simulink model "Mo_phong_3"  (R2019a)
settings: Solver=FixedStepAuto  StartTime=0.0  StopTime=55  FixedStep=0.01  RelTol=1e-3
undefined symbols (not defined in the file): magnitude
libraries: mobileRoboticsLib x13, simulink x6
settings Model: Creator=chemi  LastModifiedBy=chemi

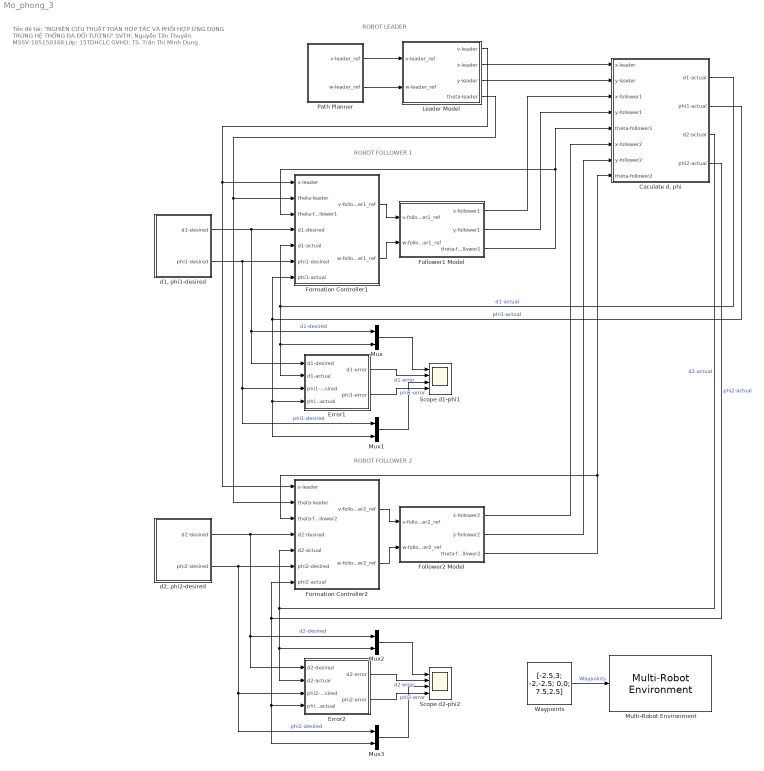
== system Mo_phong_3 ==
  note: ROBOT FOLLOWER 1
  note: ROBOT LEADER
  note: ROBOT FOLLOWER 2
  note: Tên đề tài: "NGHIÊN CỨU THUẬT TOÁN HỢP TÁC
      | VÀ PHỐI HỢP ỨNG DỤNG TRONG HỆ THỐNG
      | ĐA ĐỐI TƯỢNG"
      |
      | SVTH: Nguyễn Tấn Thuyền MSSV:105150348
      | Lớp: 15TDHCLC
      | GVHD: TS. Trần Thị Minh Dung
  "Caculate d, phi" : Subsystem
  Error1 : Subsystem
  Error2 : Subsystem
  Follower1 Model : Subsystem
  Follower2 Model : Subsystem
  Formation Controller1 : Subsystem
  Formation Controller2 : Subsystem
  Leader Model : Subsystem
  Multi-Robot Environment : mobileRoboticsLib/Environments/Multi-Robot Environment  numRobots=3  showWaypoints=on  showObjects=off  objectColors=[1 0 0;0 1 0;0 0 1]  objectMarkers='s'  showRobotIds=on  plotSensorLines=off
      settings: SourceProductName=Mobile Robotics Simulation Toolbox
  Mux{,1..3} (4 alike) : Mux  Inputs=2
  Path Planner : Subsystem
  Scope d1-phi1 : Scope  NumInputPorts=4
  Scope d2-phi2 : Scope  NumInputPorts=4
  Waypoints : Constant  Value=[-2.5,3; -2,-2.5; 0,0; 7.5,2.5]
  "d1, phi1-desired" : Subsystem
  "d2, phi2-desired" : Subsystem
  wires:
  Path Planner/1(v-leader_ref) -> Leader Model/1(v-leader_ref)
  Leader Model/2(x-leader) -> "Caculate d, phi"/1(x-leader)
  Follower1 Model/2(y-follower1) -> "Caculate d, phi"/4(y-follower1)
  Leader Model/3(y-leader) -> "Caculate d, phi"/2(y-leader)
  Follower1 Model/1(x-follower1) -> "Caculate d, phi"/3(x-follower1)
  Follower1 Model/3(theta-follower1) -> "Caculate d, phi"/5(theta-follower1), Formation Controller1/3(theta-follower1)
  "Caculate d, phi"/2(phi1-actual) -> Formation Controller1/7(phi1-actual), Mux1/2, Error1/4(phi1-actual)  "phi1-actual"
  "Caculate d, phi"/1(d1-actual) -> Formation Controller1/5(d1-actual), Mux/2, Error1/2(d1-actual)  "d1-actual"
  Leader Model/1(v-leader) -> Formation Controller1/1(v-leader), Formation Controller2/1(v-leader)
  Leader Model/4(theta-leader) -> Formation Controller1/2(theta-leader), Formation Controller2/2(theta-leader)
  "d1, phi1-desired"/2(phi1-desired) -> Mux1/1, Error1/3(phi1-desired), Formation Controller1/6(phi1-desired)  "phi1-desired"
  "d1, phi1-desired"/1(d1-desired) -> Mux/1, Error1/1(d1-desired), Formation Controller1/4(d1-desired)  "d1-desired"
  Formation Controller2/2(w-follower2_ref) -> Follower2 Model/2(w-follower2_ref)
  Follower2 Model/1(x-follower2) -> "Caculate d, phi"/6(x-follower2)
  Follower2 Model/2(y-follower2) -> "Caculate d, phi"/7(y-follower2)
  Follower2 Model/3(theta-follower2) -> "Caculate d, phi"/8(theta-follower2), Formation Controller2/3(theta-follower2)
  "Caculate d, phi"/3(d2-actual) -> Mux2/2, Error2/2(d2-actual), Formation Controller2/5(d2-actual)  "d2-actual"
  "Caculate d, phi"/4(phi2-actual) -> Formation Controller2/7(phi2-actual), Mux3/2, Error2/4(phi2-actual)  "phi2-actual"
  "d2, phi2-desired"/1(d2-desired) -> Mux2/1, Error2/1(d2-desired), Formation Controller2/4(d2-desired)  "d2-desired"
  "d2, phi2-desired"/2(phi2-desired) -> Mux3/1, Error2/3(phi2-desired), Formation Controller2/6(phi2-desired)  "phi2-desired"
  Waypoints/1 -> Multi-Robot Environment/1  "Waypoints"
  Path Planner/2(w-leader_ref) -> Leader Model/2(w-leader_ref)
  Formation Controller1/1(v-follower1_ref) -> Follower1 Model/1(v-follower1_ref)
  Formation Controller1/2(w-follower1_ref) -> Follower1 Model/2(w-follower1_ref)
  Formation Controller2/1(v-follower2_ref) -> Follower2 Model/1(v-follower2_ref)
  Mux/1 -> Scope d1-phi1/1
  Error1/1(d1-error) -> Scope d1-phi1/2  "d1-error"
  Mux1/1 -> Scope d1-phi1/3
  Error1/2(phi1-error) -> Scope d1-phi1/4  "phi1-error"
  Mux2/1 -> Scope d2-phi2/1
  Error2/1(d2-error) -> Scope d2-phi2/2  "d2-error"
  Mux3/1 -> Scope d2-phi2/3
  Error2/2(phi2-error) -> Scope d2-phi2/4  "phi2-error"

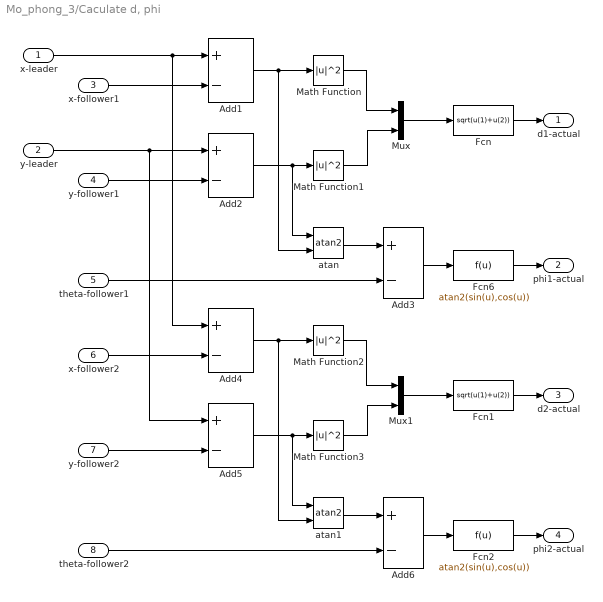
== system Mo_phong_3/Caculate d, phi ==
  x-leader : Inport
  y-leader : Inport  Port=2
  x-follower1 : Inport  Port=3
  y-follower1 : Inport  Port=4
  theta-follower1 : Inport  Port=5
  x-follower2 : Inport  Port=6
  y-follower2 : Inport  Port=7
  theta-follower2 : Inport  Port=8
  Add{1..6} (6 alike) : Sum  Inputs=+-
  Fcn : Fcn  Expr=sqrt(u(1)+u(2))
  Fcn1 : Fcn  Expr=sqrt(u(1)+u(2))
  Fcn2 : Fcn  Expr=atan2(sin(u),cos(u))
  Fcn6 : Fcn  Expr=atan2(sin(u),cos(u))
  Math Function{,1..3} (4 alike) : Math  Operator=magnitude^2  SaturateOnIntegerOverflow=on
  Mux : Mux  Inputs=2
  Mux1 : Mux  Inputs=2
  atan : Trigonometry  Operator=atan2
  atan1 : Trigonometry  Operator=atan2
  d1-actual : Outport
  phi1-actual : Outport  Port=2
  d2-actual : Outport  Port=3
  phi2-actual : Outport  Port=4
  wires:
  Math Function1/1 -> Mux/2
  Math Function/1 -> Mux/1
  Mux/1 -> Fcn/1
  Fcn/1 -> d1-actual/1
  Add2/1 -> atan/1, Math Function1/1
  Add1/1 -> atan/2, Math Function/1
  x-follower1/1 -> Add1/2
  y-follower1/1 -> Add2/2
  atan/1 -> Add3/1
  theta-follower1/1 -> Add3/2
  y-follower2/1 -> Add5/2
  y-leader/1 -> Add5/1, Add2/1
  x-follower2/1 -> Add4/2
  x-leader/1 -> Add4/1, Add1/1
  Add4/1 -> atan1/2, Math Function2/1
  Add5/1 -> atan1/1, Math Function3/1
  Fcn1/1 -> d2-actual/1
  Mux1/1 -> Fcn1/1
  Math Function2/1 -> Mux1/1
  Math Function3/1 -> Mux1/2
  atan1/1 -> Add6/1
  theta-follower2/1 -> Add6/2
  Add3/1 -> Fcn6/1
  Add6/1 -> Fcn2/1
  Fcn6/1 -> phi1-actual/1
  Fcn2/1 -> phi2-actual/1

== system Mo_phong_3/Error1 ==
  d1-desired : Inport
  d1-actual : Inport  Port=2
  phi1-desired : Inport  Port=3
  phi1-actual : Inport  Port=4
  Add2 : Sum  Inputs=+-
  Add3 : Sum  Inputs=+-
  d1-error : Outport
  phi1-error : Outport  Port=2
  wires:
  phi1-actual/1 -> Add3/2
  d1-actual/1 -> Add2/2
  phi1-desired/1 -> Add3/1
  d1-desired/1 -> Add2/1
  Add2/1 -> d1-error/1
  Add3/1 -> phi1-error/1

== system Mo_phong_3/Error2 ==
  d2-desired : Inport
  d2-actual : Inport  Port=2
  phi2-desired : Inport  Port=3
  phi2-actual : Inport  Port=4
  Add2 : Sum  Inputs=+-
  Add3 : Sum  Inputs=+-
  d2-error : Outport
  phi2-error : Outport  Port=2
  wires:
  phi2-actual/1 -> Add3/2
  d2-actual/1 -> Add2/2
  phi2-desired/1 -> Add3/1
  d2-desired/1 -> Add2/1
  Add2/1 -> d2-error/1
  Add3/1 -> phi2-error/1

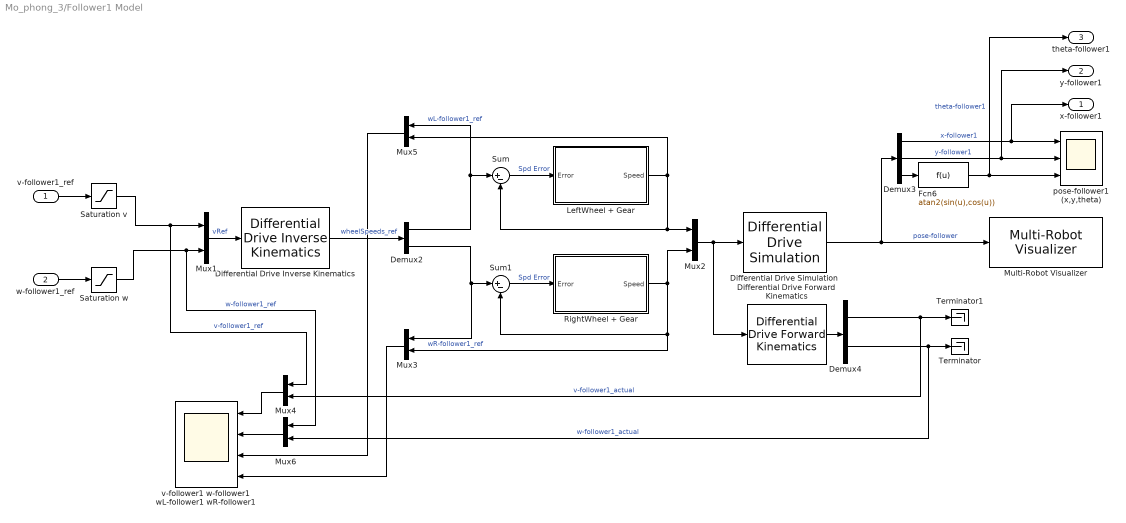
== system Mo_phong_3/Follower1 Model ==
  v-follower1_ref : Inport
  w-follower1_ref : Inport  Port=2
  Demux2 : Demux  Outputs=2
  Demux3 : Demux  Outputs=3
  Demux4 : Demux  Outputs=2
  Differential Drive Forward Kinematics : mobileRoboticsLib/Kinematic Models/Differential Drive/Differential Drive Forward Kinematics  wheelRadius=0.0425  wheelBase=0.25
      settings: SourceProductName=Mobile Robotics Simulation Toolbox
  Differential Drive Inverse Kinematics : mobileRoboticsLib/Kinematic Models/Differential Drive/Differential Drive Inverse Kinematics  wheelRadius=0.0425  wheelBase=0.25
      settings: SourceProductName=Mobile Robotics Simulation Library
  Differential Drive Simulation : mobileRoboticsLib/Kinematic Models/Differential Drive/Differential Drive Simulation  wheelRadius=0.0425  wheelBase=0.25  initX=-2.5  initY=3  initAngle=0  Ts=0.01
      settings: SourceProductName=Mobile Robotics Simulation Library
  Fcn6 : Fcn  Expr=atan2(sin(u),cos(u))
  LeftWheel + Gear : Subsystem
  Multi-Robot Visualizer : mobileRoboticsLib/Environments/Multi-Robot Visualizer  idx=2  radius=0.15  robotColor=[0.39 0.83 0.07]  showTraj=on  hasLidar=off  sensorOffset=[0,0]  scanAngles=[-pi/4, 0, pi/4]  hasObjDetector=off  objDetectorOffset=[0,0]  objDetectorAngle=0  objDetectorFOV=pi/3  objDetectorMaxRange=5
      settings: SourceProductName=Mobile Robotics Simulation Toolbox
  Mux{1..6} (6 alike) : Mux  Inputs=2
  RightWheel + Gear : Subsystem
  Saturation v : Saturate  UpperLimit=1  LowerLimit=0
  Saturation w : Saturate  UpperLimit=0.8  LowerLimit=-0.8
  Sum : Sum  Inputs=|+-
  Sum1 : Sum  Inputs=|+-
  Terminator : Terminator
  Terminator1 : Terminator
  pose-follower1 (x,y,theta) : Scope  NumInputPorts=3
  v-follower1 w-follower1 wL-follower1 wR-follower1 : Scope  NumInputPorts=4
  x-follower1 : Outport
  y-follower1 : Outport  Port=2
  theta-follower1 : Outport  Port=3
  wires:
  Demux3/2 -> pose-follower1 (x,y,theta)/2, y-follower1/1  "y-follower1"
  Differential Drive Simulation/1 -> Multi-Robot Visualizer/1, Demux3/1  "pose-follower"
  Demux3/3 -> Fcn6/1
  Differential Drive Inverse Kinematics/1 -> Demux2/1  "wheelSpeeds_ref"
  v-follower1_ref/1 -> Saturation v/1
  Demux3/1 -> pose-follower1 (x,y,theta)/1, x-follower1/1  "x-follower1"
  w-follower1_ref/1 -> Saturation w/1
  Mux1/1 -> Differential Drive Inverse Kinematics/1  "vRef"
  Demux2/2 -> Mux3/1, Sum1/1  "wR-follower1_ref"
  Demux2/1 -> Mux5/1, Sum/1  "wL-follower1_ref"
  Sum/1 -> LeftWheel + Gear/1(Error)  "Spd Error"
  LeftWheel + Gear/1(Speed) -> Mux2/1, Sum/2, Mux5/2
  Sum1/1 -> RightWheel + Gear/1(Error)  "Spd Error"
  RightWheel + Gear/1(Speed) -> Mux3/2, Sum1/2, Mux2/2
  Mux2/1 -> Differential Drive Simulation/1, Differential Drive Forward Kinematics/1
  Demux4/2 -> Mux6/2, Terminator/1  "w-follower1_actual"
  Differential Drive Forward Kinematics/1 -> Demux4/1
  Demux4/1 -> Terminator1/1, Mux4/2  "v-follower1_actual"
  Saturation v/1 -> Mux1/1, Mux4/1  "v-follower1_ref"
  Saturation w/1 -> Mux6/1, Mux1/2  "w-follower1_ref"
  Fcn6/1 -> pose-follower1 (x,y,theta)/3, theta-follower1/1  "theta-follower1"
  Mux4/1 -> v-follower1 w-follower1 wL-follower1 wR-follower1/1
  Mux6/1 -> v-follower1 w-follower1 wL-follower1 wR-follower1/2
  Mux5/1 -> v-follower1 w-follower1 wL-follower1 wR-follower1/3
  Mux3/1 -> v-follower1 w-follower1 wL-follower1 wR-follower1/4

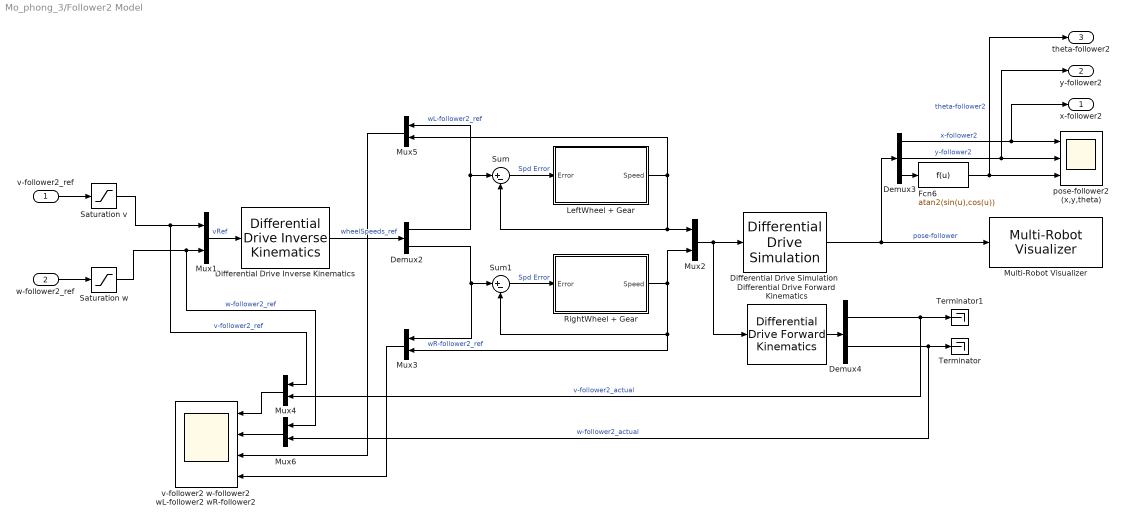
== system Mo_phong_3/Follower2 Model ==
  v-follower2_ref : Inport
  w-follower2_ref : Inport  Port=2
  Demux2 : Demux  Outputs=2
  Demux3 : Demux  Outputs=3
  Demux4 : Demux  Outputs=2
  Differential Drive Forward Kinematics : mobileRoboticsLib/Kinematic Models/Differential Drive/Differential Drive Forward Kinematics  wheelRadius=0.0425  wheelBase=0.25
      settings: SourceProductName=Mobile Robotics Simulation Toolbox
  Differential Drive Inverse Kinematics : mobileRoboticsLib/Kinematic Models/Differential Drive/Differential Drive Inverse Kinematics  wheelRadius=0.0425  wheelBase=0.25
      settings: SourceProductName=Mobile Robotics Simulation Library
  Differential Drive Simulation : mobileRoboticsLib/Kinematic Models/Differential Drive/Differential Drive Simulation  wheelRadius=0.0425  wheelBase=0.25  initX=-2  initY=-2.5  initAngle=0  Ts=0.01
      settings: SourceProductName=Mobile Robotics Simulation Library
  Fcn6 : Fcn  Expr=atan2(sin(u),cos(u))
  LeftWheel + Gear : Subsystem
  Multi-Robot Visualizer : mobileRoboticsLib/Environments/Multi-Robot Visualizer  idx=3  radius=0.15  robotColor=[0.00 0.45 0.74]  showTraj=on  hasLidar=off  sensorOffset=[0,0]  scanAngles=[-pi/4, 0, pi/4]  hasObjDetector=off  objDetectorOffset=[0,0]  objDetectorAngle=0  objDetectorFOV=pi/3  objDetectorMaxRange=5
      settings: SourceProductName=Mobile Robotics Simulation Toolbox
  Mux{1..6} (6 alike) : Mux  Inputs=2
  RightWheel + Gear : Subsystem
  Saturation v : Saturate  UpperLimit=1  LowerLimit=0
  Saturation w : Saturate  UpperLimit=0.8  LowerLimit=-0.8
  Sum : Sum  Inputs=|+-
  Sum1 : Sum  Inputs=|+-
  Terminator : Terminator
  Terminator1 : Terminator
  pose-follower2 (x,y,theta) : Scope  NumInputPorts=3
  v-follower2 w-follower2 wL-follower2 wR-follower2 : Scope  NumInputPorts=4
  x-follower2 : Outport
  y-follower2 : Outport  Port=2
  theta-follower2 : Outport  Port=3
  wires:
  Demux3/2 -> pose-follower2 (x,y,theta)/2, y-follower2/1  "y-follower2"
  Differential Drive Simulation/1 -> Multi-Robot Visualizer/1, Demux3/1  "pose-follower"
  Demux3/3 -> Fcn6/1
  Differential Drive Inverse Kinematics/1 -> Demux2/1  "wheelSpeeds_ref"
  v-follower2_ref/1 -> Saturation v/1
  Demux3/1 -> pose-follower2 (x,y,theta)/1, x-follower2/1  "x-follower2"
  w-follower2_ref/1 -> Saturation w/1
  Mux1/1 -> Differential Drive Inverse Kinematics/1  "vRef"
  Demux2/2 -> Mux3/1, Sum1/1  "wR-follower2_ref"
  Demux2/1 -> Mux5/1, Sum/1  "wL-follower2_ref"
  Sum/1 -> LeftWheel + Gear/1(Error)  "Spd Error"
  LeftWheel + Gear/1(Speed) -> Mux2/1, Sum/2, Mux5/2
  Sum1/1 -> RightWheel + Gear/1(Error)  "Spd Error"
  RightWheel + Gear/1(Speed) -> Mux3/2, Sum1/2, Mux2/2
  Mux2/1 -> Differential Drive Simulation/1, Differential Drive Forward Kinematics/1
  Demux4/2 -> Mux6/2, Terminator/1  "w-follower2_actual"
  Differential Drive Forward Kinematics/1 -> Demux4/1
  Demux4/1 -> Terminator1/1, Mux4/2  "v-follower2_actual"
  Saturation v/1 -> Mux1/1, Mux4/1  "v-follower2_ref"
  Saturation w/1 -> Mux6/1, Mux1/2  "w-follower2_ref"
  Fcn6/1 -> pose-follower2 (x,y,theta)/3, theta-follower2/1  "theta-follower2"
  Mux4/1 -> v-follower2 w-follower2 wL-follower2 wR-follower2/1
  Mux6/1 -> v-follower2 w-follower2 wL-follower2 wR-follower2/2
  Mux5/1 -> v-follower2 w-follower2 wL-follower2 wR-follower2/3
  Mux3/1 -> v-follower2 w-follower2 wL-follower2 wR-follower2/4

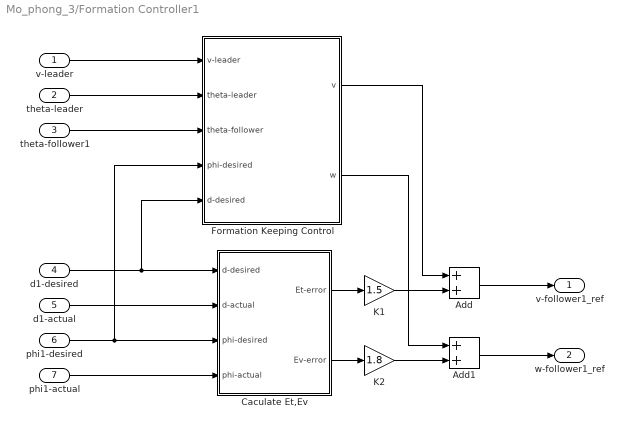
== system Mo_phong_3/Formation Controller1 ==
  v-leader : Inport
  theta-leader : Inport  Port=2
  theta-follower1 : Inport  Port=3
  d1-desired : Inport  Port=4
  d1-actual : Inport  Port=5
  phi1-desired : Inport  Port=6
  phi1-actual : Inport  Port=7
  Add : Sum
  Add1 : Sum
  Caculate Et,Ev : Subsystem
  Formation Keeping Control : Subsystem
  K1 : Gain  Gain=1.5
  K2 : Gain  Gain=1.8
  v-follower1_ref : Outport
  w-follower1_ref : Outport  Port=2
  wires:
  phi1-desired/1 -> Formation Keeping Control/4(phi-desired), Caculate Et,Ev/3(phi-desired)
  theta-follower1/1 -> Formation Keeping Control/3(theta-follower)
  Caculate Et,Ev/1(Et-error) -> K1/1
  Caculate Et,Ev/2(Ev-error) -> K2/1
  theta-leader/1 -> Formation Keeping Control/2(theta-leader)
  d1-actual/1 -> Caculate Et,Ev/2(d-actual)
  v-leader/1 -> Formation Keeping Control/1(v-leader)
  Add/1 -> v-follower1_ref/1
  phi1-actual/1 -> Caculate Et,Ev/4(phi-actual)
  Add1/1 -> w-follower1_ref/1
  d1-desired/1 -> Formation Keeping Control/5(d-desired), Caculate Et,Ev/1(d-desired)
  Formation Keeping Control/1(v) -> Add/1
  K1/1 -> Add/2
  Formation Keeping Control/2(w) -> Add1/1
  K2/1 -> Add1/2

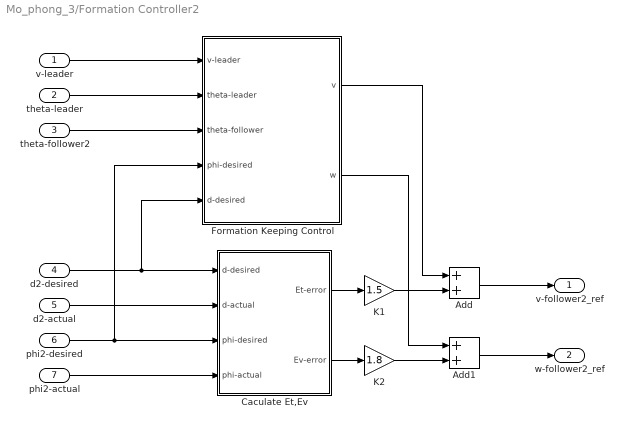
== system Mo_phong_3/Formation Controller2 ==
  v-leader : Inport
  theta-leader : Inport  Port=2
  theta-follower2 : Inport  Port=3
  d2-desired : Inport  Port=4
  d2-actual : Inport  Port=5
  phi2-desired : Inport  Port=6
  phi2-actual : Inport  Port=7
  Add : Sum
  Add1 : Sum
  Caculate Et,Ev : Subsystem
  Formation Keeping Control : Subsystem
  K1 : Gain  Gain=1.5
  K2 : Gain  Gain=1.8
  v-follower2_ref : Outport
  w-follower2_ref : Outport  Port=2
  wires:
  K2/1 -> Add1/2
  Formation Keeping Control/2(w) -> Add1/1
  K1/1 -> Add/2
  Formation Keeping Control/1(v) -> Add/1
  d2-desired/1 -> Caculate Et,Ev/1(d-desired), Formation Keeping Control/5(d-desired)
  Add1/1 -> w-follower2_ref/1
  phi2-actual/1 -> Caculate Et,Ev/4(phi-actual)
  Add/1 -> v-follower2_ref/1
  v-leader/1 -> Formation Keeping Control/1(v-leader)
  d2-actual/1 -> Caculate Et,Ev/2(d-actual)
  theta-leader/1 -> Formation Keeping Control/2(theta-leader)
  Caculate Et,Ev/2(Ev-error) -> K2/1
  Caculate Et,Ev/1(Et-error) -> K1/1
  theta-follower2/1 -> Formation Keeping Control/3(theta-follower)
  phi2-desired/1 -> Caculate Et,Ev/3(phi-desired), Formation Keeping Control/4(phi-desired)

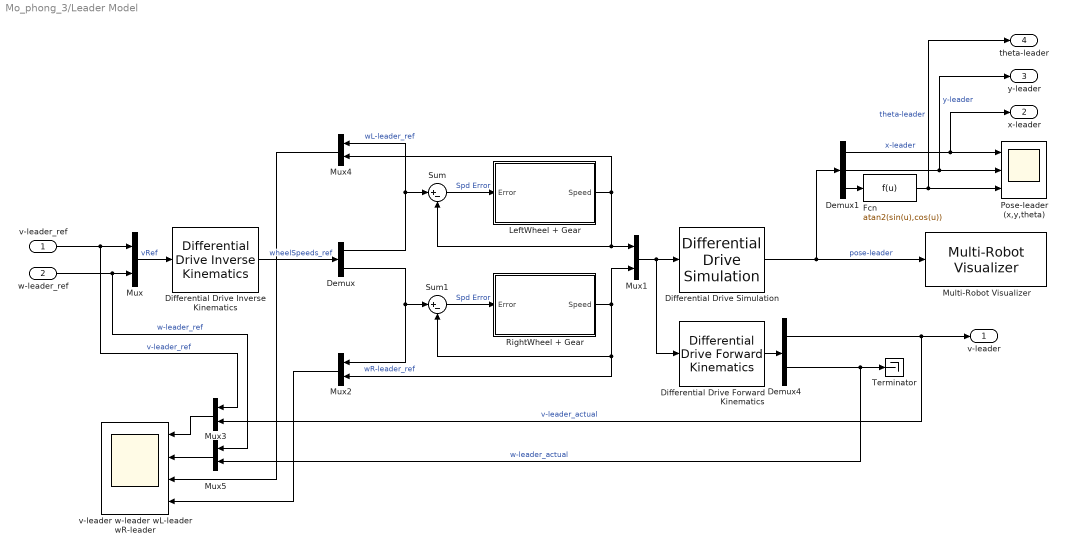
== system Mo_phong_3/Leader Model ==
  v-leader_ref : Inport
  w-leader_ref : Inport  Port=2
  Demux : Demux  Outputs=2
  Demux1 : Demux  Outputs=3
  Demux4 : Demux  Outputs=2
  Differential Drive Forward Kinematics : mobileRoboticsLib/Kinematic Models/Differential Drive/Differential Drive Forward Kinematics  wheelRadius=0.0425  wheelBase=0.25
      settings: SourceProductName=Mobile Robotics Simulation Toolbox
  Differential Drive Inverse Kinematics : mobileRoboticsLib/Kinematic Models/Differential Drive/Differential Drive Inverse Kinematics  wheelRadius=0.0425  wheelBase=0.25
      settings: SourceProductName=Mobile Robotics Simulation Toolbox
  Differential Drive Simulation : mobileRoboticsLib/Kinematic Models/Differential Drive/Differential Drive Simulation  wheelRadius=0.0425  wheelBase=0.25  initX=0  initY=0  initAngle=0  Ts=0.01
      settings: SourceProductName=Mobile Robotics Simulation Toolbox
  Fcn : Fcn  Expr=atan2(sin(u),cos(u))
  LeftWheel + Gear : Subsystem
  Multi-Robot Visualizer : mobileRoboticsLib/Environments/Multi-Robot Visualizer  idx=1  radius=0.15  robotColor=[1.00 0.41 0.16]  showTraj=on  hasLidar=off  sensorOffset=[0,0]  scanAngles=[-pi/4, 0, pi/4]  hasObjDetector=off  objDetectorOffset=[0,0]  objDetectorAngle=0  objDetectorFOV=pi/3  objDetectorMaxRange=5
      settings: SourceProductName=Mobile Robotics Simulation Toolbox
  Mux{,1..5} (6 alike) : Mux  Inputs=2
  Pose-leader (x,y,theta) : Scope  NumInputPorts=3
  RightWheel + Gear : Subsystem
  Sum : Sum  Inputs=|+-
  Sum1 : Sum  Inputs=|+-
  Terminator : Terminator
  v-leader w-leader wL-leader wR-leader : Scope  NumInputPorts=4
  v-leader : Outport
  x-leader : Outport  Port=2
  y-leader : Outport  Port=3
  theta-leader : Outport  Port=4
  wires:
  Differential Drive Inverse Kinematics/1 -> Demux/1  "wheelSpeeds_ref"
  w-leader_ref/1 -> Mux5/1, Mux/2  "w-leader_ref"
  Demux1/3 -> Fcn/1
  Differential Drive Simulation/1 -> Multi-Robot Visualizer/1, Demux1/1  "pose-leader"
  v-leader_ref/1 -> Mux/1, Mux3/1  "v-leader_ref"
  Demux1/2 -> Pose-leader (x,y,theta)/2, y-leader/1  "y-leader"
  Demux1/1 -> Pose-leader (x,y,theta)/1, x-leader/1  "x-leader"
  Demux/1 -> Mux4/1, Sum/1  "wL-leader_ref"
  Demux/2 -> Mux2/1, Sum1/1  "wR-leader_ref"
  Demux4/2 -> Mux5/2, Terminator/1  "w-leader_actual"
  Differential Drive Forward Kinematics/1 -> Demux4/1
  Mux/1 -> Differential Drive Inverse Kinematics/1  "vRef"
  Demux4/1 -> Mux3/2, v-leader/1  "v-leader_actual"
  Sum/1 -> LeftWheel + Gear/1(Error)  "Spd Error"
  LeftWheel + Gear/1(Speed) -> Sum/2, Mux1/1, Mux4/2
  Sum1/1 -> RightWheel + Gear/1(Error)  "Spd Error"
  RightWheel + Gear/1(Speed) -> Mux2/2, Sum1/2, Mux1/2
  Mux1/1 -> Differential Drive Simulation/1, Differential Drive Forward Kinematics/1
  Fcn/1 -> Pose-leader (x,y,theta)/3, theta-leader/1  "theta-leader"
  Mux3/1 -> v-leader w-leader wL-leader wR-leader/1
  Mux4/1 -> v-leader w-leader wL-leader wR-leader/3
  Mux2/1 -> v-leader w-leader wL-leader wR-leader/4
  Mux5/1 -> v-leader w-leader wL-leader wR-leader/2

== system Mo_phong_3/Path Planner ==
  Angular Speed Desired : Step  Time=15  After=0.2  SampleTime=0
  Velocity Desired : Constant  Value=0.5
  Zero-Order Hold : ZeroOrderHold  SampleTime=0.01
  Zero-Order Hold1 : ZeroOrderHold  SampleTime=0.01
  v-leader_ref : Outport
  w-leader_ref : Outport  Port=2
  wires:
  Velocity Desired/1 -> Zero-Order Hold1/1
  Zero-Order Hold/1 -> w-leader_ref/1
  Zero-Order Hold1/1 -> v-leader_ref/1
  Angular Speed Desired/1 -> Zero-Order Hold/1

== system Mo_phong_3/d1, phi1-desired ==
  d1-ref : Constant
  phi1-ref : Constant  Value=-pi/4
  d1-desired : Outport
  phi1-desired : Outport  Port=2
  wires:
  d1-ref/1 -> d1-desired/1
  phi1-ref/1 -> phi1-desired/1

== system Mo_phong_3/d2, phi2-desired ==
  d2-ref : Constant
  phi2-ref : Constant  Value=pi/4
  d2-desired : Outport
  phi2-desired : Outport  Port=2
  wires:
  phi2-ref/1 -> phi2-desired/1
  d2-ref/1 -> d2-desired/1

== system Mo_phong_3/Follower1 Model/LeftWheel + Gear ==
  Error : Inport
  DC Motor : Subsystem
  Gear : Gain  Gain=1/34
  Speed Controller : Subsystem
  Speed : Outport
  wires:
  Speed Controller/1(Control) -> DC Motor/1(Input)  "Control Input"
  DC Motor/1(Output) -> Gear/1  "Output"
  Gear/1 -> Speed/1
  Error/1 -> Speed Controller/1(Error)

== system Mo_phong_3/Follower1 Model/RightWheel + Gear ==
  Error : Inport
  DC Motor : Subsystem
  Gear : Gain  Gain=1/34
  Speed Controller : Subsystem
  Speed : Outport
  wires:
  Speed Controller/1(Control) -> DC Motor/1(Input)  "Control Input"
  DC Motor/1(Output) -> Gear/1  "Output"
  Gear/1 -> Speed/1
  Error/1 -> Speed Controller/1(Error)

== system Mo_phong_3/Follower2 Model/LeftWheel + Gear ==
  Error : Inport
  DC Motor : Subsystem
  Gear : Gain  Gain=1/34
  Speed Controller : Subsystem
  Speed : Outport
  wires:
  Speed Controller/1(Control) -> DC Motor/1(Input)  "Control Input"
  DC Motor/1(Output) -> Gear/1  "Output"
  Gear/1 -> Speed/1
  Error/1 -> Speed Controller/1(Error)

== system Mo_phong_3/Follower2 Model/RightWheel + Gear ==
  Error : Inport
  DC Motor : Subsystem
  Gear : Gain  Gain=1/34
  Speed Controller : Subsystem
  Speed : Outport
  wires:
  Speed Controller/1(Control) -> DC Motor/1(Input)  "Control Input"
  DC Motor/1(Output) -> Gear/1  "Output"
  Gear/1 -> Speed/1
  Error/1 -> Speed Controller/1(Error)

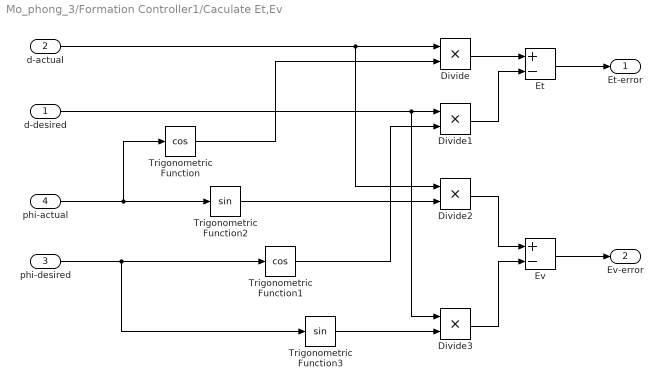
== system Mo_phong_3/Formation Controller1/Caculate Et,Ev ==
  d-desired : Inport
  d-actual : Inport  Port=2
  phi-desired : Inport  Port=3
  phi-actual : Inport  Port=4
  Divide{,1..3} (4 alike) : Product  Inputs=**
  Et : Sum  Inputs=+-
  Ev : Sum  Inputs=+-
  Trigonometric Function : Trigonometry  Operator=cos
  Trigonometric Function1 : Trigonometry  Operator=cos
  Trigonometric Function2 : Trigonometry
  Trigonometric Function3 : Trigonometry
  Et-error : Outport
  Ev-error : Outport  Port=2
  wires:
  d-desired/1 -> Divide3/1, Divide1/1
  d-actual/1 -> Divide2/1, Divide/1
  phi-desired/1 -> Trigonometric Function3/1, Trigonometric Function1/1
  phi-actual/1 -> Trigonometric Function2/1, Trigonometric Function/1
  Trigonometric Function/1 -> Divide/2
  Trigonometric Function1/1 -> Divide1/2
  Divide1/1 -> Et/2
  Divide/1 -> Et/1
  Trigonometric Function2/1 -> Divide2/2
  Trigonometric Function3/1 -> Divide3/2
  Divide3/1 -> Ev/2
  Divide2/1 -> Ev/1
  Et/1 -> Et-error/1
  Ev/1 -> Ev-error/1

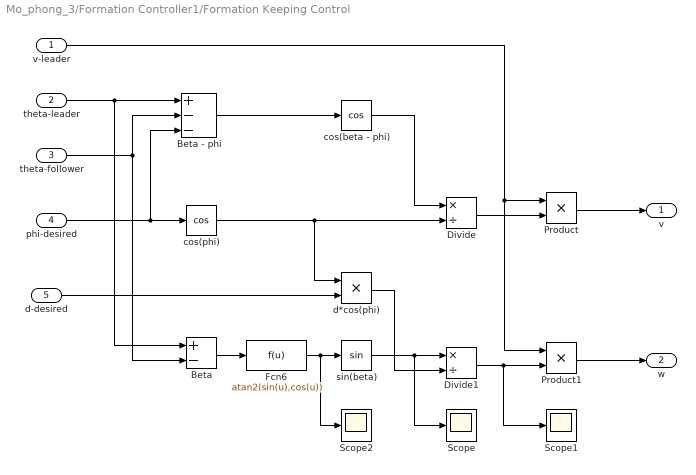
== system Mo_phong_3/Formation Controller1/Formation Keeping Control ==
  v-leader : Inport
  theta-leader : Inport  Port=2
  theta-follower : Inport  Port=3
  phi-desired : Inport  Port=4
  d-desired : Inport  Port=5
  Beta : Sum  Inputs=+-
  Beta - phi : Sum  Inputs=+--
  Divide : Product  Inputs=*/
  Divide1 : Product  Inputs=*/
  Fcn6 : Fcn  Expr=atan2(sin(u),cos(u))
  Product : Product
  Product1 : Product
  Scope : Scope
  Scope1 : Scope
  Scope2 : Scope
  cos(beta - phi) : Trigonometry  Operator=cos
  cos(phi) : Trigonometry  Operator=cos
  d*cos(phi) : Product  Inputs=**
  sin(beta) : Trigonometry
  v : Outport
  w : Outport  Port=2
  wires:
  Beta - phi/1 -> cos(beta - phi)/1
  Product/1 -> v/1
  sin(beta)/1 -> Scope/1, Divide1/1
  v-leader/1 -> Product1/1, Product/1
  cos(phi)/1 -> Divide/2, d*cos(phi)/1
  Divide1/1 -> Scope1/1, Product1/2
  Beta/1 -> Fcn6/1
  theta-leader/1 -> Beta/1, Beta - phi/1
  cos(beta - phi)/1 -> Divide/1
  Divide/1 -> Product/2
  theta-follower/1 -> Beta/2, Beta - phi/2
  Product1/1 -> w/1
  d*cos(phi)/1 -> Divide1/2
  phi-desired/1 -> cos(phi)/1, Beta - phi/3
  d-desired/1 -> d*cos(phi)/2
  Fcn6/1 -> Scope2/1, sin(beta)/1

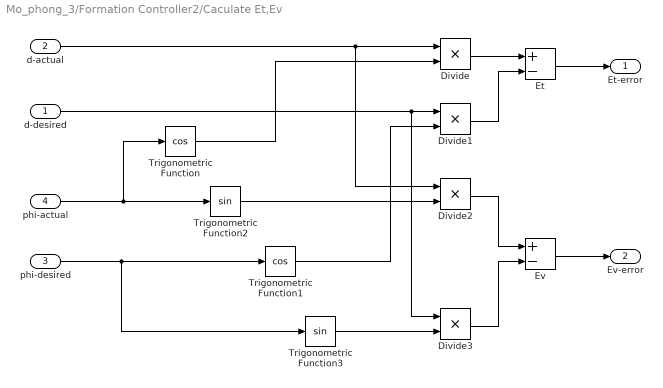
== system Mo_phong_3/Formation Controller2/Caculate Et,Ev ==
  d-desired : Inport
  d-actual : Inport  Port=2
  phi-desired : Inport  Port=3
  phi-actual : Inport  Port=4
  Divide{,1..3} (4 alike) : Product  Inputs=**
  Et : Sum  Inputs=+-
  Ev : Sum  Inputs=+-
  Trigonometric Function : Trigonometry  Operator=cos
  Trigonometric Function1 : Trigonometry  Operator=cos
  Trigonometric Function2 : Trigonometry
  Trigonometric Function3 : Trigonometry
  Et-error : Outport
  Ev-error : Outport  Port=2
  wires:
  Ev/1 -> Ev-error/1
  Et/1 -> Et-error/1
  Divide2/1 -> Ev/1
  Divide3/1 -> Ev/2
  Trigonometric Function3/1 -> Divide3/2
  Trigonometric Function2/1 -> Divide2/2
  Divide/1 -> Et/1
  Divide1/1 -> Et/2
  Trigonometric Function1/1 -> Divide1/2
  Trigonometric Function/1 -> Divide/2
  phi-actual/1 -> Trigonometric Function/1, Trigonometric Function2/1
  phi-desired/1 -> Trigonometric Function1/1, Trigonometric Function3/1
  d-actual/1 -> Divide/1, Divide2/1
  d-desired/1 -> Divide1/1, Divide3/1

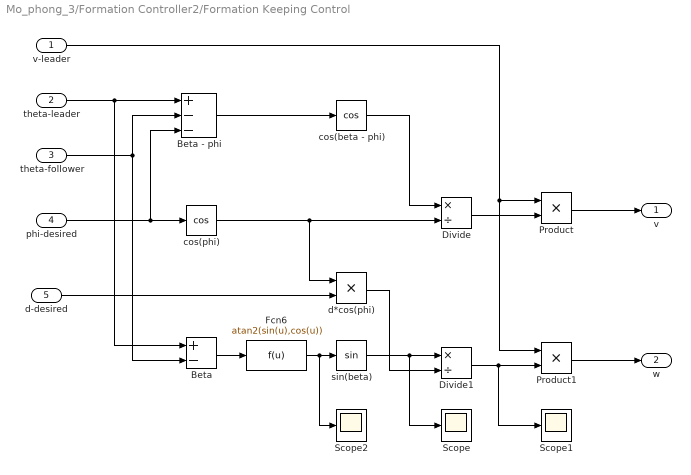
== system Mo_phong_3/Formation Controller2/Formation Keeping Control ==
  v-leader : Inport
  theta-leader : Inport  Port=2
  theta-follower : Inport  Port=3
  phi-desired : Inport  Port=4
  d-desired : Inport  Port=5
  Beta : Sum  Inputs=+-
  Beta - phi : Sum  Inputs=+--
  Divide : Product  Inputs=*/
  Divide1 : Product  Inputs=*/
  Fcn6 : Fcn  Expr=atan2(sin(u),cos(u))
  Product : Product
  Product1 : Product
  Scope : Scope
  Scope1 : Scope
  Scope2 : Scope
  cos(beta - phi) : Trigonometry  Operator=cos
  cos(phi) : Trigonometry  Operator=cos
  d*cos(phi) : Product  Inputs=**
  sin(beta) : Trigonometry
  v : Outport
  w : Outport  Port=2
  wires:
  d-desired/1 -> d*cos(phi)/2
  phi-desired/1 -> Beta - phi/3, cos(phi)/1
  d*cos(phi)/1 -> Divide1/2
  Product1/1 -> w/1
  theta-follower/1 -> Beta - phi/2, Beta/2
  Divide/1 -> Product/2
  cos(beta - phi)/1 -> Divide/1
  theta-leader/1 -> Beta - phi/1, Beta/1
  Beta/1 -> Fcn6/1
  Divide1/1 -> Product1/2, Scope1/1
  cos(phi)/1 -> d*cos(phi)/1, Divide/2
  v-leader/1 -> Product/1, Product1/1
  sin(beta)/1 -> Divide1/1, Scope/1
  Product/1 -> v/1
  Beta - phi/1 -> cos(beta - phi)/1
  Fcn6/1 -> sin(beta)/1, Scope2/1

== system Mo_phong_3/Leader Model/LeftWheel + Gear ==
  Error : Inport
  DC Motor : Subsystem
  Gear : Gain  Gain=1/34
  Speed Controller : Subsystem
  Speed : Outport
  wires:
  Speed Controller/1(Control) -> DC Motor/1(Input)  "Control Input"
  DC Motor/1(Output) -> Gear/1  "Output"
  Gear/1 -> Speed/1
  Error/1 -> Speed Controller/1(Error)

== system Mo_phong_3/Leader Model/RightWheel + Gear ==
  Error : Inport
  DC Motor : Subsystem
  Gear : Gain  Gain=1/34
  Speed Controller : Subsystem
  Speed : Outport
  wires:
  Error/1 -> Speed Controller/1(Error)
  Gear/1 -> Speed/1
  DC Motor/1(Output) -> Gear/1  "Output"
  Speed Controller/1(Control) -> DC Motor/1(Input)  "Control Input"

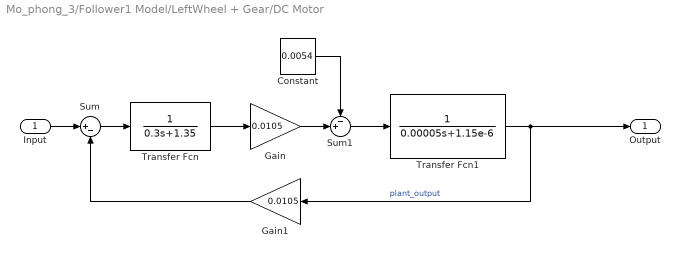
== system Mo_phong_3/Follower1 Model/LeftWheel + Gear/DC Motor ==
  Input : Inport
  Constant : Constant  Value=0.0054
  Gain : Gain  Gain=0.0105
  Gain1 : Gain  Gain=0.0105
  Sum : Sum  Inputs=|+-
  Sum1 : Sum  Inputs=-+|
  Transfer Fcn : TransferFcn  Denominator=[0.3 1.35]
  Transfer Fcn1 : TransferFcn  Denominator=[0.00005 1.15e-6]
  Output : Outport
  wires:
  Transfer Fcn1/1 -> Gain1/1, Output/1  "plant_output"
  Input/1 -> Sum/1
  Sum/1 -> Transfer Fcn/1
  Transfer Fcn/1 -> Gain/1
  Gain/1 -> Sum1/2
  Sum1/1 -> Transfer Fcn1/1
  Constant/1 -> Sum1/1
  Gain1/1 -> Sum/2

== system Mo_phong_3/Follower1 Model/LeftWheel + Gear/Speed Controller ==
  Error : Inport
  1-D Lookup Table1 : Lookup_n-D  NumberOfTableDimensions=1  BreakpointsForDimension1=[-255:1:255]  Table=[-11.999994:0.0470588:11.999994]  InternalRulePriority=Speed  RndMeth=Simplest  InputSameDT=on
  PID Controller : simulink/Continuous/PID Controller  Controller=PID  Form=Parallel  TimeDomain=Discrete-time  SampleTime=0.01  IntegratorMethod=Forward Euler  FilterMethod=Forward Euler  ControllerParametersSource=internal  P=20  I=16.75  D=4.2  UseFilter=off  N=100  TunerSelectOption=Transfer Function Based (PID Tuner App)  InitialConditionSource=internal  InitialConditionForIntegrator=0  InitialConditionForFilter=0  DifferentiatorICPrevScaledInput=0  ExternalReset=none  TrackingMode=off  Kt=1  LimitOutput=on  UpperSaturationLimit=255  LowerSaturationLimit=-255  LinearizeAsGain=on  AntiWindupMode=none  Kb=1  POutMin=[]  POutMax=[]  IOutMin=[]  IOutMax=[]  DOutMin=[]  DOutMax=[]  NOutMin=[]  NOutMax=[]  SumOutMin=[]  SumOutMax=[]  SaturationOutMin=[]  SaturationOutMax=[]  PParamMin=[]  PParamMax=[]  IParamMin=[]  IParamMax=[]  DParamMin=[]  DParamMax=[]  NParamMin=[]  NParamMax=[]  KbParamMin=[]  KbParamMax=[]  KtParamMin=[]  KtParamMax=[]  KbOutMin=[]  KbOutMax=[]  KtOutMin=[]  KtOutMax=[]  IntegratorOutMin=[]  IntegratorOutMax=[]  FilterOutMin=[]  FilterOutMax=[]  SumI1OutMin=[]  SumI1OutMax=[]  SumI2OutMin=[]  SumI2OutMax=[]  SumI3OutMin=[]  SumI3OutMax=[]  SumI4OutMin=[]  SumI4OutMax=[]  SumDOutMin=[]  SumDOutMax=[]  DifferentiatorOutMin=[]  DifferentiatorOutMax=[]  FilterDiffOutCoefMin=[]  FilterDiffOutCoefMax=[]  ReciprocalOutMin=[]  ReciprocalOutMax=[]  SumDenOutMin=[]  SumDenOutMax=[]  SumNumOutMin=[]  SumNumOutMax=[]  DivideOutMin=[]  DivideOutMax=[]  IntegratorContinuousStateAttributes=''  IntegratorStateMustResolveToSignalObject=off  IntegratorRTWStateStorageClass=Auto  FilterContinuousStateAttributes=''  FilterStateMustResolveToSignalObject=off  FilterRTWStateStorageClass=Auto  ParallelPVariant=InternalParameters  IdealPVariant=Disabled  IVariant=InternalParameters  DVariant=InternalParameters  IntegratorVariant=Discrete  SatVariant=Enabled  AWVariant=Passthrough  PCopyVariant=Disabled  TRVariant=Disabled  FdbkBlocksVariant=Forward  IdealPFdbkVariant=Disabled  SatFdbkVariant=Disabled  DerivativeFilterVariant=Differentiator  NVariant=Passthrough  NCopyVariant=Disabled_SignalSpec  FilterICVariant=InternalICsDifferentiator  IntegratorICVariant=InternalICs  ExternalResetVariant=Disabled  TRSumVariant=Passthrough  SumFdbkVariant=Disabled  SumVariant=Sum_PID
  Control : Outport
  wires:
  Error/1 -> PID Controller/1
  PID Controller/1 -> 1-D Lookup Table1/1
  1-D Lookup Table1/1 -> Control/1

== system Mo_phong_3/Follower1 Model/RightWheel + Gear/DC Motor ==
  Input : Inport
  Constant : Constant  Value=0.0054
  Gain : Gain  Gain=0.0105
  Gain1 : Gain  Gain=0.0105
  Sum : Sum  Inputs=|+-
  Sum1 : Sum  Inputs=-+|
  Transfer Fcn : TransferFcn  Denominator=[0.3 1.35]
  Transfer Fcn1 : TransferFcn  Denominator=[0.00005 1.15e-6]
  Output : Outport
  wires:
  Transfer Fcn1/1 -> Gain1/1, Output/1  "plant_output"
  Input/1 -> Sum/1
  Sum/1 -> Transfer Fcn/1
  Transfer Fcn/1 -> Gain/1
  Gain/1 -> Sum1/2
  Sum1/1 -> Transfer Fcn1/1
  Constant/1 -> Sum1/1
  Gain1/1 -> Sum/2

== system Mo_phong_3/Follower1 Model/RightWheel + Gear/Speed Controller ==
  Error : Inport
  1-D Lookup Table1 : Lookup_n-D  NumberOfTableDimensions=1  BreakpointsForDimension1=[-255:1:255]  Table=[-11.999994:0.0470588:11.999994]  InternalRulePriority=Speed  RndMeth=Simplest  InputSameDT=on
  PID Controller : simulink/Continuous/PID Controller  Controller=PID  Form=Parallel  TimeDomain=Discrete-time  SampleTime=0.01  IntegratorMethod=Forward Euler  FilterMethod=Forward Euler  ControllerParametersSource=internal  P=20  I=16.75  D=4.2  UseFilter=off  N=100  TunerSelectOption=Transfer Function Based (PID Tuner App)  InitialConditionSource=internal  InitialConditionForIntegrator=0  InitialConditionForFilter=0  DifferentiatorICPrevScaledInput=0  ExternalReset=none  TrackingMode=off  Kt=1  LimitOutput=on  UpperSaturationLimit=255  LowerSaturationLimit=-255  LinearizeAsGain=on  AntiWindupMode=none  Kb=1  POutMin=[]  POutMax=[]  IOutMin=[]  IOutMax=[]  DOutMin=[]  DOutMax=[]  NOutMin=[]  NOutMax=[]  SumOutMin=[]  SumOutMax=[]  SaturationOutMin=[]  SaturationOutMax=[]  PParamMin=[]  PParamMax=[]  IParamMin=[]  IParamMax=[]  DParamMin=[]  DParamMax=[]  NParamMin=[]  NParamMax=[]  KbParamMin=[]  KbParamMax=[]  KtParamMin=[]  KtParamMax=[]  KbOutMin=[]  KbOutMax=[]  KtOutMin=[]  KtOutMax=[]  IntegratorOutMin=[]  IntegratorOutMax=[]  FilterOutMin=[]  FilterOutMax=[]  SumI1OutMin=[]  SumI1OutMax=[]  SumI2OutMin=[]  SumI2OutMax=[]  SumI3OutMin=[]  SumI3OutMax=[]  SumI4OutMin=[]  SumI4OutMax=[]  SumDOutMin=[]  SumDOutMax=[]  DifferentiatorOutMin=[]  DifferentiatorOutMax=[]  FilterDiffOutCoefMin=[]  FilterDiffOutCoefMax=[]  ReciprocalOutMin=[]  ReciprocalOutMax=[]  SumDenOutMin=[]  SumDenOutMax=[]  SumNumOutMin=[]  SumNumOutMax=[]  DivideOutMin=[]  DivideOutMax=[]  IntegratorContinuousStateAttributes=''  IntegratorStateMustResolveToSignalObject=off  IntegratorRTWStateStorageClass=Auto  FilterContinuousStateAttributes=''  FilterStateMustResolveToSignalObject=off  FilterRTWStateStorageClass=Auto  ParallelPVariant=InternalParameters  IdealPVariant=Disabled  IVariant=InternalParameters  DVariant=InternalParameters  IntegratorVariant=Discrete  SatVariant=Enabled  AWVariant=Passthrough  PCopyVariant=Disabled  TRVariant=Disabled  FdbkBlocksVariant=Forward  IdealPFdbkVariant=Disabled  SatFdbkVariant=Disabled  DerivativeFilterVariant=Differentiator  NVariant=Passthrough  NCopyVariant=Disabled_SignalSpec  FilterICVariant=InternalICsDifferentiator  IntegratorICVariant=InternalICs  ExternalResetVariant=Disabled  TRSumVariant=Passthrough  SumFdbkVariant=Disabled  SumVariant=Sum_PID
  Control : Outport
  wires:
  Error/1 -> PID Controller/1
  PID Controller/1 -> 1-D Lookup Table1/1
  1-D Lookup Table1/1 -> Control/1

== system Mo_phong_3/Follower2 Model/LeftWheel + Gear/DC Motor ==
  Input : Inport
  Constant : Constant  Value=0.0054
  Gain : Gain  Gain=0.0105
  Gain1 : Gain  Gain=0.0105
  Sum : Sum  Inputs=|+-
  Sum1 : Sum  Inputs=-+|
  Transfer Fcn : TransferFcn  Denominator=[0.3 1.35]
  Transfer Fcn1 : TransferFcn  Denominator=[0.00005 1.15e-6]
  Output : Outport
  wires:
  Transfer Fcn1/1 -> Gain1/1, Output/1  "plant_output"
  Input/1 -> Sum/1
  Sum/1 -> Transfer Fcn/1
  Transfer Fcn/1 -> Gain/1
  Gain/1 -> Sum1/2
  Sum1/1 -> Transfer Fcn1/1
  Constant/1 -> Sum1/1
  Gain1/1 -> Sum/2

== system Mo_phong_3/Follower2 Model/LeftWheel + Gear/Speed Controller ==
  Error : Inport
  1-D Lookup Table1 : Lookup_n-D  NumberOfTableDimensions=1  BreakpointsForDimension1=[-255:1:255]  Table=[-11.999994:0.0470588:11.999994]  InternalRulePriority=Speed  RndMeth=Simplest  InputSameDT=on
  PID Controller : simulink/Continuous/PID Controller  Controller=PID  Form=Parallel  TimeDomain=Discrete-time  SampleTime=0.01  IntegratorMethod=Forward Euler  FilterMethod=Forward Euler  ControllerParametersSource=internal  P=20  I=16.75  D=4.2  UseFilter=off  N=100  TunerSelectOption=Transfer Function Based (PID Tuner App)  InitialConditionSource=internal  InitialConditionForIntegrator=0  InitialConditionForFilter=0  DifferentiatorICPrevScaledInput=0  ExternalReset=none  TrackingMode=off  Kt=1  LimitOutput=on  UpperSaturationLimit=255  LowerSaturationLimit=-255  LinearizeAsGain=on  AntiWindupMode=none  Kb=1  POutMin=[]  POutMax=[]  IOutMin=[]  IOutMax=[]  DOutMin=[]  DOutMax=[]  NOutMin=[]  NOutMax=[]  SumOutMin=[]  SumOutMax=[]  SaturationOutMin=[]  SaturationOutMax=[]  PParamMin=[]  PParamMax=[]  IParamMin=[]  IParamMax=[]  DParamMin=[]  DParamMax=[]  NParamMin=[]  NParamMax=[]  KbParamMin=[]  KbParamMax=[]  KtParamMin=[]  KtParamMax=[]  KbOutMin=[]  KbOutMax=[]  KtOutMin=[]  KtOutMax=[]  IntegratorOutMin=[]  IntegratorOutMax=[]  FilterOutMin=[]  FilterOutMax=[]  SumI1OutMin=[]  SumI1OutMax=[]  SumI2OutMin=[]  SumI2OutMax=[]  SumI3OutMin=[]  SumI3OutMax=[]  SumI4OutMin=[]  SumI4OutMax=[]  SumDOutMin=[]  SumDOutMax=[]  DifferentiatorOutMin=[]  DifferentiatorOutMax=[]  FilterDiffOutCoefMin=[]  FilterDiffOutCoefMax=[]  ReciprocalOutMin=[]  ReciprocalOutMax=[]  SumDenOutMin=[]  SumDenOutMax=[]  SumNumOutMin=[]  SumNumOutMax=[]  DivideOutMin=[]  DivideOutMax=[]  IntegratorContinuousStateAttributes=''  IntegratorStateMustResolveToSignalObject=off  IntegratorRTWStateStorageClass=Auto  FilterContinuousStateAttributes=''  FilterStateMustResolveToSignalObject=off  FilterRTWStateStorageClass=Auto  ParallelPVariant=InternalParameters  IdealPVariant=Disabled  IVariant=InternalParameters  DVariant=InternalParameters  IntegratorVariant=Discrete  SatVariant=Enabled  AWVariant=Passthrough  PCopyVariant=Disabled  TRVariant=Disabled  FdbkBlocksVariant=Forward  IdealPFdbkVariant=Disabled  SatFdbkVariant=Disabled  DerivativeFilterVariant=Differentiator  NVariant=Passthrough  NCopyVariant=Disabled_SignalSpec  FilterICVariant=InternalICsDifferentiator  IntegratorICVariant=InternalICs  ExternalResetVariant=Disabled  TRSumVariant=Passthrough  SumFdbkVariant=Disabled  SumVariant=Sum_PID
  Control : Outport
  wires:
  Error/1 -> PID Controller/1
  PID Controller/1 -> 1-D Lookup Table1/1
  1-D Lookup Table1/1 -> Control/1

== system Mo_phong_3/Follower2 Model/RightWheel + Gear/DC Motor ==
  Input : Inport
  Constant : Constant  Value=0.0054
  Gain : Gain  Gain=0.0105
  Gain1 : Gain  Gain=0.0105
  Sum : Sum  Inputs=|+-
  Sum1 : Sum  Inputs=-+|
  Transfer Fcn : TransferFcn  Denominator=[0.3 1.35]
  Transfer Fcn1 : TransferFcn  Denominator=[0.00005 1.15e-6]
  Output : Outport
  wires:
  Transfer Fcn1/1 -> Gain1/1, Output/1  "plant_output"
  Input/1 -> Sum/1
  Sum/1 -> Transfer Fcn/1
  Transfer Fcn/1 -> Gain/1
  Gain/1 -> Sum1/2
  Sum1/1 -> Transfer Fcn1/1
  Constant/1 -> Sum1/1
  Gain1/1 -> Sum/2

== system Mo_phong_3/Follower2 Model/RightWheel + Gear/Speed Controller ==
  Error : Inport
  1-D Lookup Table1 : Lookup_n-D  NumberOfTableDimensions=1  BreakpointsForDimension1=[-255:1:255]  Table=[-11.999994:0.0470588:11.999994]  InternalRulePriority=Speed  RndMeth=Simplest  InputSameDT=on
  PID Controller : simulink/Continuous/PID Controller  Controller=PID  Form=Parallel  TimeDomain=Discrete-time  SampleTime=0.01  IntegratorMethod=Forward Euler  FilterMethod=Forward Euler  ControllerParametersSource=internal  P=20  I=16.75  D=4.2  UseFilter=off  N=100  TunerSelectOption=Transfer Function Based (PID Tuner App)  InitialConditionSource=internal  InitialConditionForIntegrator=0  InitialConditionForFilter=0  DifferentiatorICPrevScaledInput=0  ExternalReset=none  TrackingMode=off  Kt=1  LimitOutput=on  UpperSaturationLimit=255  LowerSaturationLimit=-255  LinearizeAsGain=on  AntiWindupMode=none  Kb=1  POutMin=[]  POutMax=[]  IOutMin=[]  IOutMax=[]  DOutMin=[]  DOutMax=[]  NOutMin=[]  NOutMax=[]  SumOutMin=[]  SumOutMax=[]  SaturationOutMin=[]  SaturationOutMax=[]  PParamMin=[]  PParamMax=[]  IParamMin=[]  IParamMax=[]  DParamMin=[]  DParamMax=[]  NParamMin=[]  NParamMax=[]  KbParamMin=[]  KbParamMax=[]  KtParamMin=[]  KtParamMax=[]  KbOutMin=[]  KbOutMax=[]  KtOutMin=[]  KtOutMax=[]  IntegratorOutMin=[]  IntegratorOutMax=[]  FilterOutMin=[]  FilterOutMax=[]  SumI1OutMin=[]  SumI1OutMax=[]  SumI2OutMin=[]  SumI2OutMax=[]  SumI3OutMin=[]  SumI3OutMax=[]  SumI4OutMin=[]  SumI4OutMax=[]  SumDOutMin=[]  SumDOutMax=[]  DifferentiatorOutMin=[]  DifferentiatorOutMax=[]  FilterDiffOutCoefMin=[]  FilterDiffOutCoefMax=[]  ReciprocalOutMin=[]  ReciprocalOutMax=[]  SumDenOutMin=[]  SumDenOutMax=[]  SumNumOutMin=[]  SumNumOutMax=[]  DivideOutMin=[]  DivideOutMax=[]  IntegratorContinuousStateAttributes=''  IntegratorStateMustResolveToSignalObject=off  IntegratorRTWStateStorageClass=Auto  FilterContinuousStateAttributes=''  FilterStateMustResolveToSignalObject=off  FilterRTWStateStorageClass=Auto  ParallelPVariant=InternalParameters  IdealPVariant=Disabled  IVariant=InternalParameters  DVariant=InternalParameters  IntegratorVariant=Discrete  SatVariant=Enabled  AWVariant=Passthrough  PCopyVariant=Disabled  TRVariant=Disabled  FdbkBlocksVariant=Forward  IdealPFdbkVariant=Disabled  SatFdbkVariant=Disabled  DerivativeFilterVariant=Differentiator  NVariant=Passthrough  NCopyVariant=Disabled_SignalSpec  FilterICVariant=InternalICsDifferentiator  IntegratorICVariant=InternalICs  ExternalResetVariant=Disabled  TRSumVariant=Passthrough  SumFdbkVariant=Disabled  SumVariant=Sum_PID
  Control : Outport
  wires:
  Error/1 -> PID Controller/1
  PID Controller/1 -> 1-D Lookup Table1/1
  1-D Lookup Table1/1 -> Control/1

== system Mo_phong_3/Leader Model/LeftWheel + Gear/DC Motor ==
  Input : Inport
  Constant : Constant  Value=0.0054
  Js+b : TransferFcn  Denominator=[0.00005 1.15e-6]
  Kb : Gain  Gain=0.0105
  Km : Gain  Gain=0.0105
  Ls+R : TransferFcn  Denominator=[0.3 1.35]
  Sum : Sum  Inputs=|+-
  Sum1 : Sum  Inputs=-+|
  Output : Outport
  wires:
  Js+b/1 -> Kb/1, Output/1
  Input/1 -> Sum/1
  Sum/1 -> Ls+R/1
  Ls+R/1 -> Km/1
  Km/1 -> Sum1/2
  Sum1/1 -> Js+b/1
  Constant/1 -> Sum1/1
  Kb/1 -> Sum/2

== system Mo_phong_3/Leader Model/LeftWheel + Gear/Speed Controller ==
  Error : Inport
  1-D Lookup Table1 : Lookup_n-D  NumberOfTableDimensions=1  BreakpointsForDimension1=[-255:1:255]  Table=[-11.999994:0.0470588:11.999994]  InternalRulePriority=Speed  RndMeth=Simplest  InputSameDT=on
  PID Controller : simulink/Continuous/PID Controller  Controller=PID  Form=Parallel  TimeDomain=Discrete-time  SampleTime=0.01  IntegratorMethod=Forward Euler  FilterMethod=Forward Euler  ControllerParametersSource=internal  P=25  I=24  D=5  UseFilter=off  N=100  TunerSelectOption=Transfer Function Based (PID Tuner App)  InitialConditionSource=internal  InitialConditionForIntegrator=0  InitialConditionForFilter=0  DifferentiatorICPrevScaledInput=0  ExternalReset=none  TrackingMode=off  Kt=1  LimitOutput=on  UpperSaturationLimit=255  LowerSaturationLimit=-255  LinearizeAsGain=on  AntiWindupMode=none  Kb=1  POutMin=[]  POutMax=[]  IOutMin=[]  IOutMax=[]  DOutMin=[]  DOutMax=[]  NOutMin=[]  NOutMax=[]  SumOutMin=[]  SumOutMax=[]  SaturationOutMin=[]  SaturationOutMax=[]  PParamMin=[]  PParamMax=[]  IParamMin=[]  IParamMax=[]  DParamMin=[]  DParamMax=[]  NParamMin=[]  NParamMax=[]  KbParamMin=[]  KbParamMax=[]  KtParamMin=[]  KtParamMax=[]  KbOutMin=[]  KbOutMax=[]  KtOutMin=[]  KtOutMax=[]  IntegratorOutMin=[]  IntegratorOutMax=[]  FilterOutMin=[]  FilterOutMax=[]  SumI1OutMin=[]  SumI1OutMax=[]  SumI2OutMin=[]  SumI2OutMax=[]  SumI3OutMin=[]  SumI3OutMax=[]  SumI4OutMin=[]  SumI4OutMax=[]  SumDOutMin=[]  SumDOutMax=[]  DifferentiatorOutMin=[]  DifferentiatorOutMax=[]  FilterDiffOutCoefMin=[]  FilterDiffOutCoefMax=[]  ReciprocalOutMin=[]  ReciprocalOutMax=[]  SumDenOutMin=[]  SumDenOutMax=[]  SumNumOutMin=[]  SumNumOutMax=[]  DivideOutMin=[]  DivideOutMax=[]  IntegratorContinuousStateAttributes=''  IntegratorStateMustResolveToSignalObject=off  IntegratorRTWStateStorageClass=Auto  FilterContinuousStateAttributes=''  FilterStateMustResolveToSignalObject=off  FilterRTWStateStorageClass=Auto  ParallelPVariant=InternalParameters  IdealPVariant=Disabled  IVariant=InternalParameters  DVariant=InternalParameters  IntegratorVariant=Discrete  SatVariant=Enabled  AWVariant=Passthrough  PCopyVariant=Disabled  TRVariant=Disabled  FdbkBlocksVariant=Forward  IdealPFdbkVariant=Disabled  SatFdbkVariant=Disabled  DerivativeFilterVariant=Differentiator  NVariant=Passthrough  NCopyVariant=Disabled_SignalSpec  FilterICVariant=InternalICsDifferentiator  IntegratorICVariant=InternalICs  ExternalResetVariant=Disabled  TRSumVariant=Passthrough  SumFdbkVariant=Disabled  SumVariant=Sum_PID
  Control : Outport
  wires:
  Error/1 -> PID Controller/1
  PID Controller/1 -> 1-D Lookup Table1/1
  1-D Lookup Table1/1 -> Control/1

== system Mo_phong_3/Leader Model/RightWheel + Gear/DC Motor ==
  Input : Inport
  Constant : Constant  Value=0.0054
  Gain : Gain  Gain=0.0105
  Gain1 : Gain  Gain=0.0105
  Sum : Sum  Inputs=|+-
  Sum1 : Sum  Inputs=-+|
  Transfer Fcn : TransferFcn  Denominator=[0.3 1.35]
  Transfer Fcn1 : TransferFcn  Denominator=[0.00005 1.15e-6]
  Output : Outport
  wires:
  Gain1/1 -> Sum/2
  Constant/1 -> Sum1/1
  Sum1/1 -> Transfer Fcn1/1
  Gain/1 -> Sum1/2
  Transfer Fcn/1 -> Gain/1
  Sum/1 -> Transfer Fcn/1
  Input/1 -> Sum/1
  Transfer Fcn1/1 -> Output/1, Gain1/1  "plant_output"

== system Mo_phong_3/Leader Model/RightWheel + Gear/Speed Controller ==
  Error : Inport
  1-D Lookup Table1 : Lookup_n-D  NumberOfTableDimensions=1  BreakpointsForDimension1=[-255:1:255]  Table=[-11.999994:0.0470588:11.999994]  InternalRulePriority=Speed  RndMeth=Simplest  InputSameDT=on
  PID Controller : simulink/Continuous/PID Controller  Controller=PID  Form=Parallel  TimeDomain=Discrete-time  SampleTime=0.01  IntegratorMethod=Forward Euler  FilterMethod=Forward Euler  ControllerParametersSource=internal  P=25  I=24  D=5  UseFilter=off  N=100  TunerSelectOption=Transfer Function Based (PID Tuner App)  InitialConditionSource=internal  InitialConditionForIntegrator=0  InitialConditionForFilter=0  DifferentiatorICPrevScaledInput=0  ExternalReset=none  TrackingMode=off  Kt=1  LimitOutput=on  UpperSaturationLimit=255  LowerSaturationLimit=-255  LinearizeAsGain=on  AntiWindupMode=none  Kb=1  POutMin=[]  POutMax=[]  IOutMin=[]  IOutMax=[]  DOutMin=[]  DOutMax=[]  NOutMin=[]  NOutMax=[]  SumOutMin=[]  SumOutMax=[]  SaturationOutMin=[]  SaturationOutMax=[]  PParamMin=[]  PParamMax=[]  IParamMin=[]  IParamMax=[]  DParamMin=[]  DParamMax=[]  NParamMin=[]  NParamMax=[]  KbParamMin=[]  KbParamMax=[]  KtParamMin=[]  KtParamMax=[]  KbOutMin=[]  KbOutMax=[]  KtOutMin=[]  KtOutMax=[]  IntegratorOutMin=[]  IntegratorOutMax=[]  FilterOutMin=[]  FilterOutMax=[]  SumI1OutMin=[]  SumI1OutMax=[]  SumI2OutMin=[]  SumI2OutMax=[]  SumI3OutMin=[]  SumI3OutMax=[]  SumI4OutMin=[]  SumI4OutMax=[]  SumDOutMin=[]  SumDOutMax=[]  DifferentiatorOutMin=[]  DifferentiatorOutMax=[]  FilterDiffOutCoefMin=[]  FilterDiffOutCoefMax=[]  ReciprocalOutMin=[]  ReciprocalOutMax=[]  SumDenOutMin=[]  SumDenOutMax=[]  SumNumOutMin=[]  SumNumOutMax=[]  DivideOutMin=[]  DivideOutMax=[]  IntegratorContinuousStateAttributes=''  IntegratorStateMustResolveToSignalObject=off  IntegratorRTWStateStorageClass=Auto  FilterContinuousStateAttributes=''  FilterStateMustResolveToSignalObject=off  FilterRTWStateStorageClass=Auto  ParallelPVariant=InternalParameters  IdealPVariant=Disabled  IVariant=InternalParameters  DVariant=InternalParameters  IntegratorVariant=Discrete  SatVariant=Enabled  AWVariant=Passthrough  PCopyVariant=Disabled  TRVariant=Disabled  FdbkBlocksVariant=Forward  IdealPFdbkVariant=Disabled  SatFdbkVariant=Disabled  DerivativeFilterVariant=Differentiator  NVariant=Passthrough  NCopyVariant=Disabled_SignalSpec  FilterICVariant=InternalICsDifferentiator  IntegratorICVariant=InternalICs  ExternalResetVariant=Disabled  TRSumVariant=Passthrough  SumFdbkVariant=Disabled  SumVariant=Sum_PID
  Control : Outport
  wires:
  1-D Lookup Table1/1 -> Control/1
  PID Controller/1 -> 1-D Lookup Table1/1
  Error/1 -> PID Controller/1
